simulink model "doppio_int"  (R2018b)
settings: Solver=VariableStepAuto  StartTime=0.0  StopTime=30  RelTol=1e-3
settings Model: Creator=Dan  LastModifiedBy=Dan

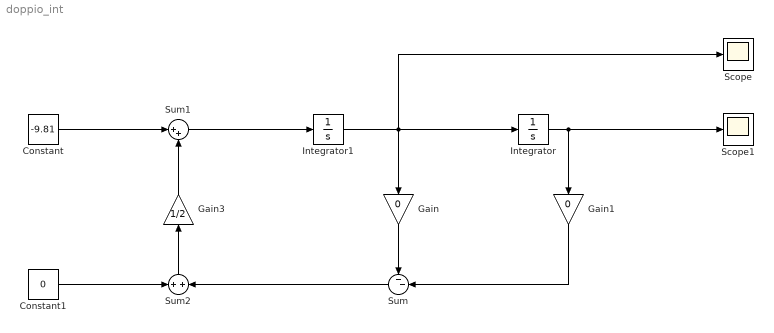
== system doppio_int ==
  Constant : Constant  Value=-9.81
  Constant1 : Constant  Value=0
  Gain : Gain  Gain=0
  Gain1 : Gain  Gain=0
  Gain3 : Gain  Gain=1/2
  Integrator : Integrator  InitialCondition=10
  Integrator1 : Integrator
  Scope : Scope
  Scope1 : Scope
  Sum : Sum  Inputs=--|
  Sum1 : Sum  Inputs=|++
  Sum2 : Sum  Inputs=+|+
  wires:
  Integrator/1 -> Scope1/1, Gain1/1
  Constant/1 -> Sum1/1
  Integrator1/1 -> Integrator/1, Scope/1, Gain/1
  Gain1/1 -> Sum/2
  Gain/1 -> Sum/1
  Sum/1 -> Sum2/2
  Sum1/1 -> Integrator1/1
  Gain3/1 -> Sum1/2
  Sum2/1 -> Gain3/1
  Constant1/1 -> Sum2/1
